simulink model "F16AeroCoefficientsModelTestHarness"  (R2024a)
settings: configuration reference "standardSILConfiguraitonParams" (kept outside this file)
undefined symbols (not defined in the file): CL, CM, CN, CX, dLdAil, dLdRud, dNdAil, dNdRud, m2ft, maxAilDefl_deg, maxRudderDefl_deg, vehicleParams
libraries: simulink_extras x1
settings Model: Creator=jerem  LastModifiedBy=jerem
settings ConfigSetRef: SourceName=standardSILConfiguraitonParams  SourceLocation=Base Workspace

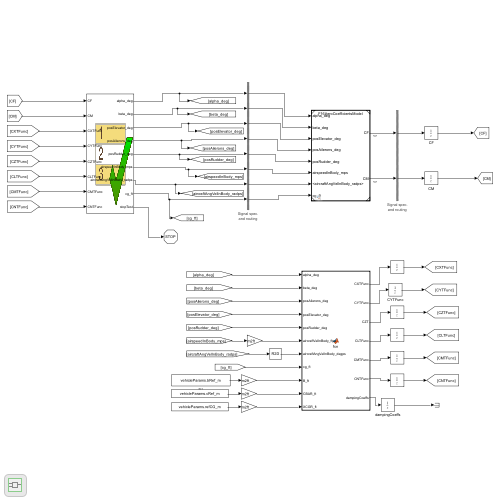
[thumbnail: Simulink's stored preview of the top-level diagram]
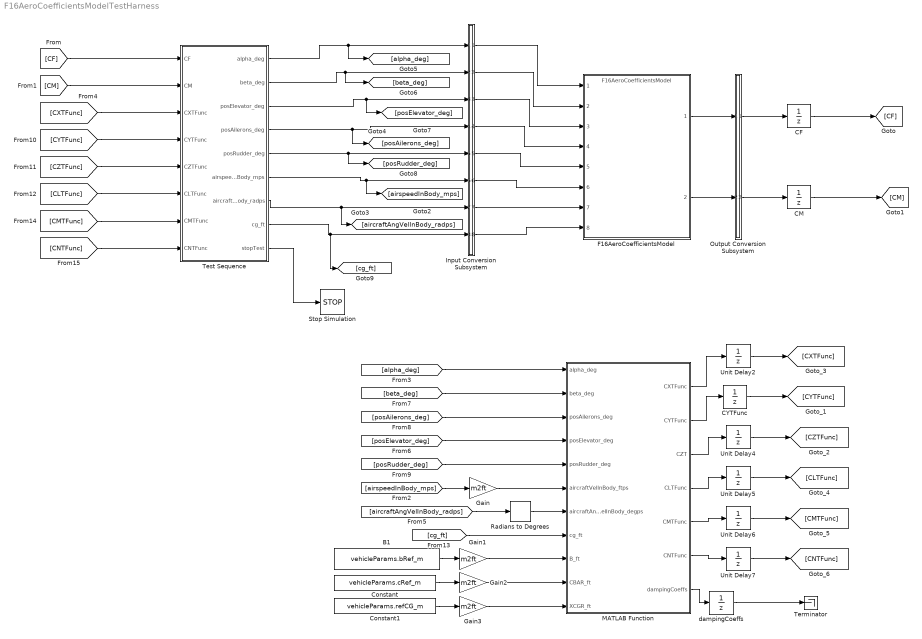
== system F16AeroCoefficientsModelTestHarness ==
  B1 : Constant  Value=vehicleParams.bRef_m
  CF : UnitDelay  SampleTime=-1  HasFrameUpgradeWarning=on
  CM : UnitDelay  SampleTime=-1  HasFrameUpgradeWarning=on
  CYTFunc : UnitDelay  SampleTime=-1  HasFrameUpgradeWarning=on
  Constant : Constant  Value=vehicleParams.cRef_m
  Constant1 : Constant  Value=vehicleParams.refCG_m
  F16AeroCoefficientsModel : ModelReference  ModelNameDialog=F16AeroCoefficientsModel  SimulationMode=Normal  ModelReferenceVersion=1.66
  Gain{,1..3} (4 alike) : Gain  Gain=m2ft
  Input Conversion Subsystem : Subsystem  Tag=__SLT_ICS__  Description=|
      | Signal spec.
      | and routing
      settings: AttributesFormatString=%<Description>
  MATLAB Function : MATLAB Function  TreatAsAtomicUnit=on
  Output Conversion Subsystem : Subsystem  Tag=__SLT_OCS__  Description=|
      | Signal spec.
      | and routing
      settings: AttributesFormatString=%<Description>
  Radians to Degrees : simulink_extras/Transformations/Radians to Degrees
  Stop Simulation : Stop
  Terminator : Terminator
  Test Sequence : Test Sequence  TreatAsAtomicUnit=on
  Unit Delay{2,4..7} (5 alike) : UnitDelay  SampleTime=-1  HasFrameUpgradeWarning=on
  dampingCoeffs : UnitDelay  SampleTime=-1  HasFrameUpgradeWarning=on
  wires:
  Output Conversion Subsystem/1(Outport_1) -> CF/1
  Output Conversion Subsystem/2(Outport_2) -> CM/1
  Input Conversion Subsystem/1(Outport_1) -> F16AeroCoefficientsModel/1
  Input Conversion Subsystem/2(Outport_2) -> F16AeroCoefficientsModel/2
  Input Conversion Subsystem/3(Outport_3) -> F16AeroCoefficientsModel/3
  Input Conversion Subsystem/4(Outport_4) -> F16AeroCoefficientsModel/4
  Input Conversion Subsystem/5(Outport_5) -> F16AeroCoefficientsModel/5
  Input Conversion Subsystem/6(Outport_6) -> F16AeroCoefficientsModel/6
  Input Conversion Subsystem/7(Outport_7) -> F16AeroCoefficientsModel/7
  Input Conversion Subsystem/8(Outport_8) -> F16AeroCoefficientsModel/8
  F16AeroCoefficientsModel/1 -> Output Conversion Subsystem/1(Inport_1)
  F16AeroCoefficientsModel/2 -> Output Conversion Subsystem/2(Inport_2)
  Gain/1 -> MATLAB Function/6(aircraftVelInBody_ftps)
  MATLAB Function/7(dampingCoeffs) -> dampingCoeffs/1
  Radians to Degrees/1 -> MATLAB Function/7(aircraftAngVelInBody_degps)
  Unit Delay7/1 -> [CNTFunc]
  dampingCoeffs/1 -> Terminator/1
  [alpha_deg] -> MATLAB Function/1(alpha_deg)
  MATLAB Function/2(CYTFunc) -> CYTFunc/1
  Unit Delay6/1 -> [CMTFunc]
  Unit Delay5/1 -> [CLTFunc]
  [posAilerons_deg] -> MATLAB Function/3(posAilerons_deg)
  MATLAB Function/4(CLTFunc) -> Unit Delay5/1
  MATLAB Function/5(CMTFunc) -> Unit Delay6/1
  MATLAB Function/3(CZT) -> Unit Delay4/1
  [posElevator_deg] -> MATLAB Function/4(posElevator_deg)
  [aircraftAngVelInBody_radps] -> Radians to Degrees/1
  MATLAB Function/6(CNTFunc) -> Unit Delay7/1
  [posRudder_deg] -> MATLAB Function/5(posRudder_deg)
  MATLAB Function/1(CXTFunc) -> Unit Delay2/1
  [beta_deg] -> MATLAB Function/2(beta_deg)
  CYTFunc/1 -> [CYTFunc]
  Unit Delay2/1 -> [CXTFunc]
  Unit Delay4/1 -> [CZTFunc]
  [airspeedInBody_mps] -> Gain/1
  CF/1 -> [CF]
  CM/1 -> [CM]
  Test Sequence/4(posAilerons_deg) -> Input Conversion Subsystem/4(Inport_4), [posAilerons_deg]
  [CF] -> Test Sequence/1(CF)
  [CYTFunc] -> Test Sequence/4(CYTFunc)
  [CNTFunc] -> Test Sequence/8(CNTFunc)
  [CMTFunc] -> Test Sequence/7(CMTFunc)
  [CZTFunc] -> Test Sequence/5(CZTFunc)
  Test Sequence/1(alpha_deg) -> Input Conversion Subsystem/1(Inport_1), [alpha_deg]
  [CXTFunc] -> Test Sequence/3(CXTFunc)
  [CM] -> Test Sequence/2(CM)
  Test Sequence/9(stopTest) -> Stop Simulation/1
  Test Sequence/6(airspeedInBody_mps) -> Input Conversion Subsystem/6(Inport_6), [airspeedInBody_mps]
  Test Sequence/5(posRudder_deg) -> Input Conversion Subsystem/5(Inport_5), [posRudder_deg]
  Test Sequence/7(aircraftAngVelInBody_radps) -> Input Conversion Subsystem/7(Inport_7), [aircraftAngVelInBody_radps]
  Test Sequence/2(beta_deg) -> Input Conversion Subsystem/2(Inport_2), [beta_deg]
  Test Sequence/8(cg_ft) -> Input Conversion Subsystem/8(Inport_8), [cg_ft]
  Test Sequence/3(posElevator_deg) -> Input Conversion Subsystem/3(Inport_3), [posElevator_deg]
  [CLTFunc] -> Test Sequence/6(CLTFunc)
  [cg_ft] -> MATLAB Function/8(cg_ft)
  Gain1/1 -> MATLAB Function/9(B_ft)
  B1/1 -> Gain1/1
  Constant/1 -> Gain2/1
  Gain2/1 -> MATLAB Function/10(CBAR_ft)
  Constant1/1 -> Gain3/1
  Gain3/1 -> MATLAB Function/11(XCGR_ft)

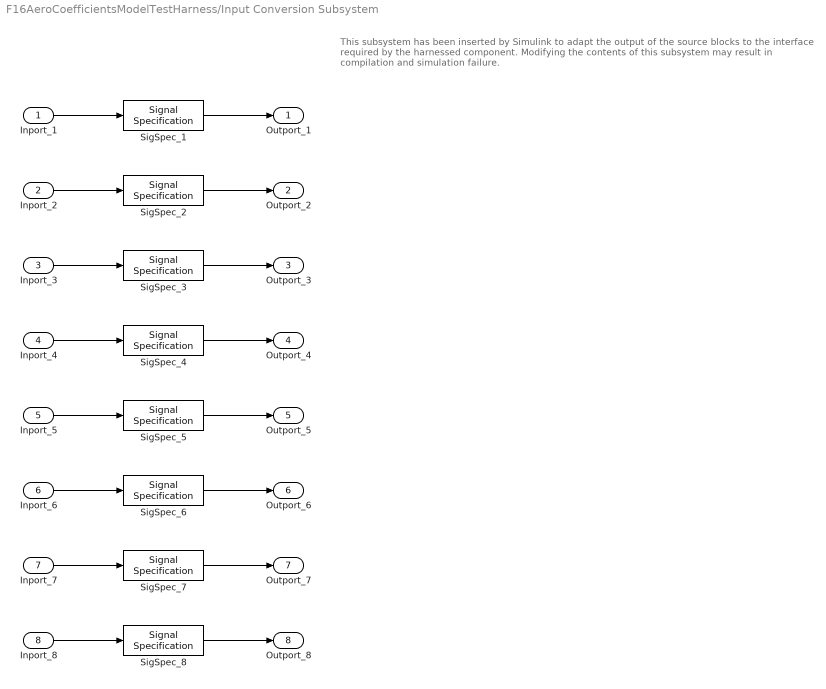
== system F16AeroCoefficientsModelTestHarness/Input Conversion Subsystem ==
  note: This subsystem has been inserted by Simulink to adapt the output of the source blocks to the interface required by the harnessed component.
      |  Modifying the contents of this subsystem may result in compilation and simulation failure.
  Inport_1 : Inport
  Inport_2 : Inport  Port=2
  Inport_3 : Inport  Port=3
  Inport_4 : Inport  Port=4
  Inport_5 : Inport  Port=5
  Inport_6 : Inport  Port=6
  Inport_7 : Inport  Port=7
  Inport_8 : Inport  Port=8
  SigSpec_{1..5} (5 alike) : SignalSpecification  OutDataTypeStr=double  Dimensions=[1]  SampleTime=0.004
  SigSpec_6 : SignalSpecification  OutDataTypeStr=double  Dimensions=[3]  SampleTime=0.004
  SigSpec_7 : SignalSpecification  OutDataTypeStr=double  Dimensions=[3]  SampleTime=0.004
  SigSpec_8 : SignalSpecification  OutDataTypeStr=double  Dimensions=[3]  SampleTime=0.004
  Outport_1 : Outport
  Outport_2 : Outport  Port=2
  Outport_3 : Outport  Port=3
  Outport_4 : Outport  Port=4
  Outport_5 : Outport  Port=5
  Outport_6 : Outport  Port=6
  Outport_7 : Outport  Port=7
  Outport_8 : Outport  Port=8
  wires:
  SigSpec_1/1 -> Outport_1/1
  Inport_1/1 -> SigSpec_1/1
  SigSpec_2/1 -> Outport_2/1
  Inport_2/1 -> SigSpec_2/1
  SigSpec_3/1 -> Outport_3/1
  Inport_3/1 -> SigSpec_3/1
  SigSpec_4/1 -> Outport_4/1
  Inport_4/1 -> SigSpec_4/1
  SigSpec_5/1 -> Outport_5/1
  Inport_5/1 -> SigSpec_5/1
  SigSpec_6/1 -> Outport_6/1
  Inport_6/1 -> SigSpec_6/1
  SigSpec_7/1 -> Outport_7/1
  Inport_7/1 -> SigSpec_7/1
  SigSpec_8/1 -> Outport_8/1
  Inport_8/1 -> SigSpec_8/1

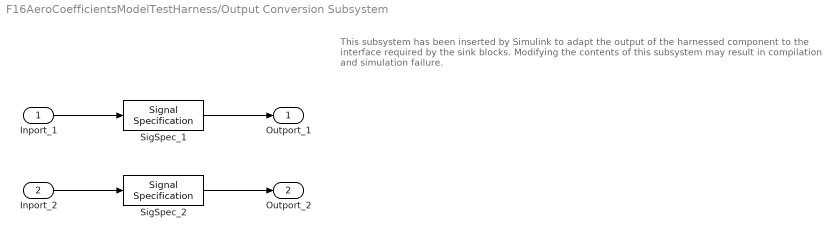
== system F16AeroCoefficientsModelTestHarness/Output Conversion Subsystem ==
  note: This subsystem has been inserted by Simulink to adapt the output of the harnessed component to the interface required by the sink blocks.
      |  Modifying the contents of this subsystem may result in compilation and simulation failure.
  Inport_1 : Inport
  Inport_2 : Inport  Port=2
  SigSpec_1 : SignalSpecification  OutDataTypeStr=double  Dimensions=[3]  SampleTime=0.004
  SigSpec_2 : SignalSpecification  OutDataTypeStr=double  Dimensions=[3]  SampleTime=0.004
  Outport_1 : Outport
  Outport_2 : Outport  Port=2
  wires:
  Inport_1/1 -> SigSpec_1/1
  SigSpec_1/1 -> Outport_1/1
  Inport_2/1 -> SigSpec_2/1
  SigSpec_2/1 -> Outport_2/1

== matlab function F16AeroCoefficientsModelTestHarness/MATLAB Function ==
  data: alpha_deg input; beta_deg input; posAilerons_deg input; posElevator_deg input; posRudder_deg input; aircraftVelInBody_ftps input; CXTFunc output; aircraftAngVelInBody_degps input; maxAilDefl_deg parameter; maxRudderDefl_deg parameter; CYTFunc output; CZT output; CLTFunc output; dNdAil parameter; dNdRud parameter; dLdRud parameter; cg_ft input; CM parameter; CMTFunc output; CN parameter; CNTFunc output; dampingCoeffs output; CX parameter; CL parameter; dLdAil parameter; B_ft input; CBAR_ft input; XCGR_ft input
function [CXTFunc, CYTFunc, CZT, CLTFunc, CMTFunc, CNTFunc, dampingCoeffs] = fcn(alpha_deg, beta_deg, posAilerons_deg, posElevator_deg, posRudder_deg, aircraftVelInBody_ftps, aircraftAngVelInBody_degps, maxAilDefl_deg, maxRudderDefl_deg, dNdAil, dNdRud, dLdRud, cg_ft, CM, CN, CX, CL, dLdAil, B_ft, CBAR_ft, XCGR_ft)

P = aircraftAngVelInBody_degps(1);
Q = aircraftAngVelInBody_degps(2);
R = aircraftAngVelInBody_degps(3);

CXFuncOutput = 0;
CZFuncOutput = 0;
DNDAOut = 0;
DNDROut = 0;
DLDAOut = 0;
DLDROut = 0;
CMT = 0;
CNOut = 0;
CLOut = 0;
dampingCoeffs = zeros(1,9);

coder.extrinsic("CXCMFunc") 
coder.extrinsic("DAMP")
coder.extrinsic("CZFunc")
coder.extrinsic("CSFunc")
coder.extrinsic("CLCNFunc")

% Other calcualtions
airspeedFreestream_ftps = aircraftVelInBody_ftps(1)^2 + aircraftVelInBody_ftps(2)^2 + aircraftVelInBody_ftps(3)^2;
VT = sqrt(airspeedFreestream_ftps);
TVT = 0.5 / VT ;
if airspeedFreestream_ftps ==0
    TVT = 0;
end
B2V = B_ft * TVT;
CQ = CBAR_ft * Q * TVT;

%Damping Coefficients
dampingCoeffs = DAMP(alpha_deg);

% CXCalcuation
CXFuncOutput  = CXCMFunc(alpha_deg, posElevator_deg, CX);
CXTFunc = CXFuncOutput + CQ * dampingCoeffs(1);

% CY Calculation
CY = -.02 * beta_deg + .021 * (posAilerons_deg / maxAilDefl_deg) + 0.086 * (posRudder_deg / maxRudderDefl_deg);
CYTFunc = CY + B2V * (dampingCoeffs(2) * R + dampingCoeffs(3) * P);

% CZ Calculation
CZFuncOutput = CZFunc(alpha_deg ,beta_deg , posElevator_deg);
CZT = CZFuncOutput + CQ * dampingCoeffs(4);

% CLT 
DAIL = posAilerons_deg / maxAilDefl_deg;
DRDR = posRudder_deg / maxRudderDefl_deg;

DNDAOut = CSFunc(alpha_deg, beta_deg, dNdAil);
DNDROut = CSFunc(alpha_deg, beta_deg, dNdRud);
DLDAOut = CSFunc(alpha_deg, beta_deg, dLdAil);
DLDROut = CSFunc(alpha_deg, beta_deg, dLdRud);
CLOut = CLCNFunc(alpha_deg, beta_deg, CL);
CLT = CLOut + DLDAOut * DAIL + DLDROut * DRDR;
CLTFunc = CLT + B2V * (dampingCoeffs(5) * R + dampingCoeffs(6) * P);

% CMT
CMT = CXCMFunc(alpha_deg, posElevator_deg, CM);
CMTFunc = CMT + CQ * dampingCoeffs(7) + CZT * (XCGR_ft(1) - cg_ft(1));

% CNT
CNOut = CLCNFunc(alpha_deg, beta_deg, CN);
CNT = CNOut + DNDAOut * DAIL + DNDROut * DRDR;
CNTFunc = CNT + B2V * (dampingCoeffs(8) * R + dampingCoeffs(9) * P) - CYTFunc * (XCGR_ft(1) - cg_ft(1)) * CBAR_ft / B_ft;

== stateflow chart F16AeroCoefficientsModelTestHarness/Test Sequence ==
  state initialization
    alpha_deg=0;
    beta_deg=0;
    posElevator_deg=0;
    posAilerons_deg=0;
    posRudder_deg=0;
    airspeedInBody_mps = zeros(3,1);
    aircraftAngVelInBody_radps = zeros(3,1);
    cg_ft = [11.32 * .35; 0; 0];
    stopTest = false;
  state verifyInitialization
    verify(isClose(CF(1), CXTFunc));
    verify(isClose(CF(2), CYTFunc));
    verify(isClose(CF(3), CZTFunc));
    verify(isClose(CM(1), CLTFunc));
    verify(isClose(CM(2), CMTFunc));
    verify(isClose(CM(3), CNTFunc));
  state airspeedIncrease
    airspeedInBody_mps(1) = 257;
  state verifyAirspeedIncrease
    verify(isClose(CF(1), CXTFunc));
    verify(isClose(CF(2), CYTFunc));
    verify(isClose(CF(3), CZTFunc));
    verify(isClose(CM(1), CLTFunc));
    verify(isClose(CM(2), CMTFunc));
    verify(isClose(CM(3), CNTFunc));
  state addSideslip
    airspeedInBody_mps(2) = 40;
    beta_deg = 3;
  state verifySideslipAdd
    verify(isClose(CF(1), CXTFunc));
    verify(isClose(CF(2), CYTFunc));
    verify(isClose(CF(3), CZTFunc));
    verify(isClose(CM(1), CLTFunc));
    verify(isClose(CM(2), CMTFunc));
    verify(isClose(CM(3), CNTFunc));
  state addCSDeflection
    posElevator_deg=5;
    posAilerons_deg=-3;
    posRudder_deg=5;
  state verifyAddCSDeflection
    verify(isClose(CF(1), CXTFunc,'atol',0.001));
    verify(isClose(CF(2), CYTFunc,'atol',0.001));
    verify(isClose(CF(3), CZTFunc,'atol',0.001));
    verify(isClose(CM(1), CLTFunc,'atol',0.001));
    verify(isClose(CM(2), CMTFunc,'atol',0.001));
    verify(isClose(CM(3), CNTFunc,'atol',0.001));
  state addAngularVelocity
    aircraftAngVelInBody_radps = [ 0.2; 0.1; 0.5];
  state verifyAddAngVel
    verify(isClose(CF(1), CXTFunc));
    verify(isClose(CF(2), CYTFunc));
    verify(isClose(CF(3), CZTFunc));
    verify(isClose(CM(1), CLTFunc));
    verify(isClose(CM(2), CMTFunc));
    verify(isClose(CM(3), CNTFunc));
  state addExtras
    airspeedInBody_mps(3) = -90;
    alpha_deg = 3;
  state verifyExtras
    verify(isClose(CF(1), CXTFunc));
    verify(isClose(CF(2), CYTFunc));
    verify(isClose(CF(3), CZTFunc));
    verify(isClose(CM(1), CLTFunc));
    verify(isClose(CM(2), CMTFunc));
    verify(isClose(CM(3), CNTFunc));
  state End
    stopTest = true;
  (default) -> initialization
  initialization -> verifyInitialization : [
      | after(3,sec)
      | ]
  verifyInitialization -> airspeedIncrease : [
      | after(2,sec)
      | ]
  airspeedIncrease -> verifyAirspeedIncrease : [
      | after(2,sec)
      | ]
  verifyAirspeedIncrease -> addSideslip : [
      | after(1,sec)
      | ]
  addSideslip -> verifySideslipAdd : [
      | after(2,sec)
      | ]
  verifySideslipAdd -> addCSDeflection : [
      | after(1,sec)
      | ]
  addCSDeflection -> verifyAddCSDeflection : [
      | after(2,sec)
      | ]
  verifyAddCSDeflection -> addAngularVelocity : [
      | after(1,sec)
      | ]
  addAngularVelocity -> verifyAddAngVel : [
      | after(2,sec)
      | ]
  verifyAddAngVel -> addExtras : [
      | after(1,sec)
      | ]
  addExtras -> verifyExtras : [
      | after(2,sec)
      | ]
  verifyExtras -> End : [
      | after(3,sec)
      | ]
  data: CF input; CM input; alpha_deg output; beta_deg output; posElevator_deg output; posAilerons_deg output; posRudder_deg output; airspeedInBody_mps output; aircraftAngVelInBody_radps output; cg_ft output; stopTest output; CXTFunc input; CYTFunc input; CZTFunc input; CLTFunc input; CMTFunc input; CNTFunc input
